simulink model "DeratingControl"  (R2021b)
settings: Solver=VariableStepAuto  StartTime=0.0  StopTime=2  FixedStep=Ts  RelTol=1e-3
model workspace (MAT data in the model file):
  df = Simulink.Parameter
  df.Value = 0.9
  df.DataType = 'auto'
  df.Complexity = 'real'
  df.Dimensions = [1 1]
undefined symbols (not defined in the file or in its folder): const_facInvTempDera, const_facMotTempDera, const_facPwrDera, const_SCD_tqDeraGenOvrd_C, const_stDera, const_tiTaskFast, const_tqBattDeraGenLim, const_tqBattDeraMotLim, const_tqDeraGen, const_tqDeraMot, const_tqDeraMotOvrd_C, const_tqEmMaxNp1, const_tqInvTempDeraMax, const_tqInvTempDeraMin, const_tqMotTempDeraMax, const_tqMotTempDeraMin, const_tqSpLim, const_tqSpLimMax, const_tqSpLimMin, const_tqTqReq
libraries: hdlsllib x10, simulink x4, mcbcontrolslib x1
settings Model: PacingRate=0.350000  Creator=win  LastModifiedBy=win

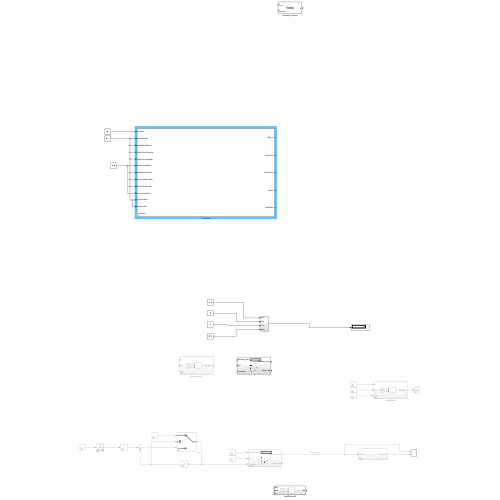
[thumbnail: Simulink's stored preview of the top-level diagram]
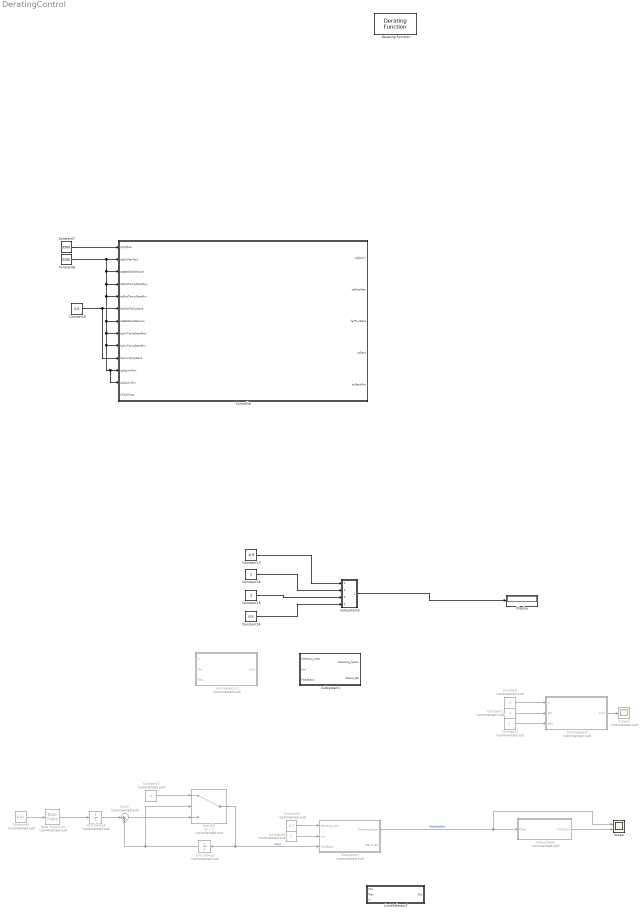
== system DeratingControl ==
  Constant : Constant  Commented=on  Value=-2
  Constant1 : Constant  Commented=on  Value=-1
  Constant13 : Constant  Value=-0.9
  Constant14 : Constant  Value=0.9
  Constant15 : Constant  Value=3
  Constant16 : Constant
  Constant2 : Constant  Commented=on
  Constant3 : Constant  Commented=on  Value=-2
  Constant4 : Constant  Commented=on
  Constant5 : Constant  Commented=on  Value=0.7
  Constant6 : Constant  Commented=on  Value=0.01
  Constant7 : Constant  Value=3500  OutDataTypeStr=int32
  Constant8 : Constant  Value=3200  OutDataTypeStr=int32
  Constant9 : Constant  Value=0.5  OutDataTypeStr=int32
  Controller : Subsystem  Description=Torque setpoint limit maximum value  mask{facGrdLimrUlim_C=50000, facGrdLimrLlim_C=-50000, bDeraMotOvrdActv_C=off, tqDeraMotOvrd_C=0, bDeraGenOvrdActv_C=off, SCD_tqDeraGenOvrd_C=0}
      mask prompts: facGrdLimrUlim_C "Gradient limiter upper factor"; facGrdLimrLlim_C "Gradient limiter lower factor"; bDeraMotOvrdActv_C "Motor mode derating override active"; tqDeraMotOvrd_C "Motor mode derating override torque"; bDeraGenOvrdActv_C "Generator mode derating override active"; SCD_tqDeraGenOvrd_C "Generator mode derating override torque"
  Derating Function : mcbcontrolslib/Derating Function  x=0.9
      settings: SourceProductBaseCode=MT
  Display : Display
  LimitSelector : Subsystem  Commented=on
  LimitSelector1 : Subsystem  Commented=on
  LimitSelector2 : Subsystem
  Rate Transition : RateTransition  Commented=on  OutPortSampleTime=1/36000000
  Scope : Scope  NumInputPorts=2
  Scope1 : Scope  Commented=on
  Subsystem : Subsystem  Commented=on
  Subsystem1 : Subsystem
  Subsystem2 : Subsystem  Commented=on
  Subsystem3 : Subsystem
  Sum1 : Sum  Commented=on  Inputs=|++
  Switch2 : Switch  Commented=on  Criteria=u2 > Threshold  Threshold=2
  Unit Delay2 : UnitDelay  Commented=on  SampleTime=-1  HasFrameUpgradeWarning=on
  Unit Delay3 : UnitDelay  Commented=on  SampleTime=-1  HasFrameUpgradeWarning=on
  wires:
  Unit Delay2/1 -> Switch2/2, Sum1/2
  Constant3/1 -> Switch2/1
  Sum1/1 -> Switch2/3
  Unit Delay3/1 -> Sum1/1
  Switch2/1 -> Subsystem/3(Feedback), Unit Delay2/1  "input"
  Constant4/1 -> Subsystem/2(Lim)
  Constant5/1 -> Subsystem/1(Derating_ratio)
  Subsystem/1(Derating_factor) -> Scope/1, Subsystem2/1(Ratio)  "DeratingOut"
  Subsystem2/1(PWM_Out) -> Scope/2
  Constant6/1 -> Rate Transition/1
  Rate Transition/1 -> Unit Delay3/1
  Constant/1 -> LimitSelector/1(In)
  Constant1/1 -> LimitSelector/2(Min)
  Constant2/1 -> LimitSelector/3(Max)
  LimitSelector/1(Limit) -> Scope1/1
  Constant8/1 -> Controller/3(tqBattDeraMotLim), Controller/4("tqMotTempDeraMax "), Controller/5("tqMotTempDeraMin "), Controller/7(tqBattDeraGenLim), Controller/8(tqInvTempDeraMax), Controller/9(tqInvTempDeraMin), Controller/11("tqSpLimMax "), Controller/12("tqSpLimMin "), Controller/2("tqEmMaxNp1 ")
  Constant7/1 -> Controller/1("tqTqReq ")
  Constant14/1 -> Subsystem3/4(Max)
  Constant13/1 -> Subsystem3/1(Min)
  Constant16/1 -> Subsystem3/2(Sat)
  Constant15/1 -> Subsystem3/3(Live)
  Subsystem3/1(Out1) -> Display/1
  Constant9/1 -> Controller/10("facInvTempDera "), Controller/6("facMotTempDera ")

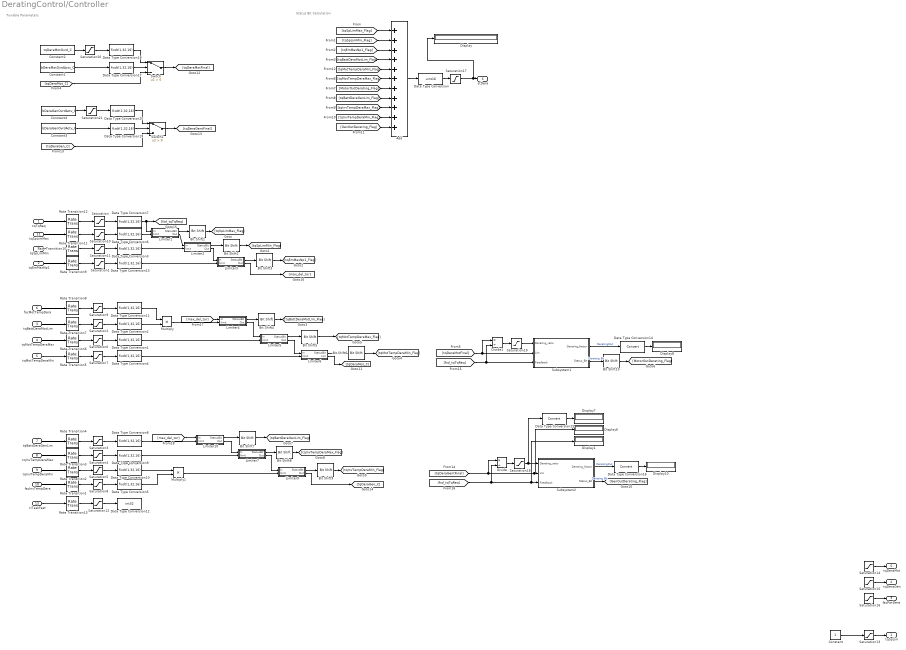
== system DeratingControl/Controller ==
  note: Tunable Parameters
  note: Status Bit Calculation
  "tqTqReq " : Inport  Description=Torque request  OutMin=const_tqTqReq(1)  OutMax=const_tqTqReq(2)  OutDataTypeStr=int32
  "tqEmMaxNp1 " : Inport  Description=EM Maximum torque N+1 step  Port=2  OutMin=const_tqEmMaxNp1(1)  OutMax=const_tqEmMaxNp1(2)  OutDataTypeStr=int32
  tqBattDeraMotLim : Inport  Description=Derated motor mode torque output according to battery limits  Port=3  OutMin=const_tqBattDeraMotLim(1)  OutMax=const_tqBattDeraMotLim(2)  OutDataTypeStr=int32
  "tqMotTempDeraMax " : Inport  Description=Derated torque maximum value according to motor temperature  Port=4  OutMin=const_tqMotTempDeraMax(1)  OutMax=const_tqMotTempDeraMax(2)  OutDataTypeStr=int32
  "tqMotTempDeraMin " : Inport  Description=Derated torque minimum value according to motor temperature  Port=5  OutMin=const_tqMotTempDeraMin(1)  OutMax=const_tqMotTempDeraMin(2)  OutDataTypeStr=int32
  "facMotTempDera " : Inport  Description=Torque derating factor according to motor temperature  Port=6  OutMin=const_facMotTempDera(1)  OutMax=const_facMotTempDera(2)  OutDataTypeStr=int32
  tqBattDeraGenLim : Inport  Description=Derated generator mode torque output according to battery limits  Port=7  OutMin=const_tqBattDeraGenLim(1)  OutMax=const_tqBattDeraGenLim(2)  OutDataTypeStr=int32
  tqInvTempDeraMax : Inport  Description=Derated torque maximum value according to inverter temperature  Port=8  OutMin=const_tqInvTempDeraMax(1)  OutMax=const_tqInvTempDeraMax(2)  OutDataTypeStr=int32
  tqInvTempDeraMin : Inport  Description=Derated torque minimum value according to inverter temperature  Port=9  OutMin=const_tqInvTempDeraMin(1)  OutMax=const_tqInvTempDeraMin(2)  OutDataTypeStr=int32
  "facInvTempDera " : Inport  Description=Torque derating factor according to inverter temperature  Port=10  OutMin=const_facInvTempDera(1)  OutMax=const_facInvTempDera(2)  OutDataTypeStr=int32
  "tqSpLimMax " : Inport  Description=Torque setpoint limit maximum value  Port=11  OutMin=const_tqSpLimMax(1)  OutMax=const_tqSpLimMax(2)  OutDataTypeStr=int32
  "tqSpLimMin " : Inport  Description=Torque setpoint limit minimum value  Port=12  OutMin=const_tqSpLimMin(1)  OutMax=const_tqSpLimMin(2)  OutDataTypeStr=int32
  "tiTaskFast " : Inport  Description=Time for the fast task (PWM task)  Port=13  OutMin=const_tiTaskFast(1)  OutMax=const_tiTaskFast(2)  OutDataTypeStr=int32
  Add : Sum  Inputs=+++++++++++
  Bit Shift1 : hdlsllib/Logic and Bit Operations/Bit Shift  mode=Shift Left Logical  N=0
  Bit Shift10 : hdlsllib/Logic and Bit Operations/Bit Shift  mode=Shift Left Logical  N=6
  Bit Shift2 : hdlsllib/Logic and Bit Operations/Bit Shift  mode=Shift Left Logical  N=1
  Bit Shift3 : hdlsllib/Logic and Bit Operations/Bit Shift  mode=Shift Left Logical  N=2
  Bit Shift4 : hdlsllib/Logic and Bit Operations/Bit Shift  mode=Shift Left Logical  N=3
  Bit Shift5 : hdlsllib/Logic and Bit Operations/Bit Shift  mode=Shift Left Logical  N=4
  Bit Shift6 : hdlsllib/Logic and Bit Operations/Bit Shift  mode=Shift Left Logical  N=5
  Bit Shift7 : hdlsllib/Logic and Bit Operations/Bit Shift  mode=Shift Left Logical  N=7
  Bit Shift8 : hdlsllib/Logic and Bit Operations/Bit Shift  mode=Shift Left Logical  N=8
  Bit Shift9 : hdlsllib/Logic and Bit Operations/Bit Shift  mode=Shift Left Logical  N=9
  Constant : Constant
  Constant1 : Constant  Value=bDeraMotOvrdActv_C
  Constant2 : Constant  Value=tqDeraMotOvrd_C
  Constant3 : Constant  Value=bDeraGenOvrdActv_C
  Constant4 : Constant  Value=bDeraGenOvrdActv_C
  Data Type Conversion : DataTypeConversion  OutDataTypeStr=uint16
  Data Type Conversion{1..11,13,17..20} (16 alike) : DataTypeConversion  OutDataTypeStr=fixdt(1,32,16)
  Data Type Conversion12 : DataTypeConversion  OutDataTypeStr=int32
  Data Type Conversion14 : DataTypeConversion
  Data Type Conversion15 : DataTypeConversion
  Data Type Conversion16 : DataTypeConversion
  Display{,1,6..8,10} (6 alike) : Display
      Display settings: Format=binary (Stored Integer)
  Divide : Product  Inputs=*/  OutDataTypeStr=fixdt(1,32,16)
  Divide1 : Product  Inputs=*/  OutDataTypeStr=fixdt(1,32,16)
  Limiter1 : Subsystem
  Limiter10 : Subsystem
  Limiter2 : Subsystem
  Limiter3 : Subsystem
  Limiter4 : Subsystem
  Limiter5 : Subsystem
  Limiter6 : Subsystem
  Limiter7 : Subsystem
  Limiter9 : Subsystem
  Multiply : Product  Inputs=**
  Multiply1 : Product  Inputs=**
  Rate Transition{1..13} (13 alike) : RateTransition  OutPortSampleTime=Ts
  Saturation : Saturate  UpperLimit=const_tqTqReq(2)  LowerLimit=const_tqTqReq(1)
  Saturation1 : Saturate  UpperLimit=const_tqEmMaxNp1(2)  LowerLimit=const_tqEmMaxNp1(1)
  Saturation10 : Saturate  UpperLimit=const_tqSpLimMax(2)  LowerLimit=const_tqSpLimMax(1)  OutDataTypeStr=int32
  Saturation11 : Saturate  UpperLimit=const_tqSpLimMin(2)  LowerLimit=const_tqSpLimMin(1)  OutDataTypeStr=int32
  Saturation12 : Saturate  UpperLimit=const_tiTaskFast(2)  LowerLimit=const_tiTaskFast(1)  OutDataTypeStr=int32
  Saturation13 : Saturate  UpperLimit=const_tqSpLim(2)  LowerLimit=const_tqSpLim(1)  OutDataTypeStr=int32
  Saturation14 : Saturate  UpperLimit=const_tqDeraMot(2)  LowerLimit=const_tqDeraMot(1)
  Saturation15 : Saturate  UpperLimit=const_tqDeraGen(2)  LowerLimit=const_tqDeraGen(1)
  Saturation16 : Saturate  UpperLimit=const_facPwrDera(2)  LowerLimit=const_facPwrDera(1)
  Saturation17 : Saturate  UpperLimit=const_stDera(2)  LowerLimit=const_stDera(1)  OutDataTypeStr=uint16
  Saturation18 : Saturate  UpperLimit=1  LowerLimit=0  OutDataTypeStr=fixdt(1,32,16)
  Saturation19 : Saturate  UpperLimit=1  LowerLimit=0  OutDataTypeStr=fixdt(1,32,16)
  Saturation2 : Saturate  UpperLimit=const_tqBattDeraMotLim(2)  LowerLimit=const_tqBattDeraMotLim(1)
  Saturation20 : Saturate  UpperLimit=const_tqDeraMotOvrd_C(2)  LowerLimit=const_tqDeraMotOvrd_C(1)  OutDataTypeStr=int32
  Saturation21 : Saturate  UpperLimit=const_SCD_tqDeraGenOvrd_C(2)  LowerLimit=const_SCD_tqDeraGenOvrd_C(1)  OutDataTypeStr=int32
  Saturation3 : Saturate  UpperLimit=const_tqBattDeraGenLim(2)  LowerLimit=const_tqBattDeraGenLim(1)
  Saturation4 : Saturate  UpperLimit=const_tqInvTempDeraMax(2)  LowerLimit=const_tqInvTempDeraMax(1)  OutDataTypeStr=int32
  Saturation5 : Saturate  UpperLimit=const_tqInvTempDeraMin(2)  LowerLimit=const_tqInvTempDeraMin(1)  OutDataTypeStr=int32
  Saturation6 : Saturate  UpperLimit=const_tqMotTempDeraMax(2)  LowerLimit=const_tqMotTempDeraMax(1)  OutDataTypeStr=int32
  Saturation7 : Saturate  UpperLimit=const_tqMotTempDeraMin(2)  LowerLimit=const_tqMotTempDeraMin(1)  OutDataTypeStr=int32
  Saturation8 : Saturate  UpperLimit=1  LowerLimit=0  OutDataTypeStr=int32
  Saturation9 : Saturate  UpperLimit=const_facMotTempDera(2)  LowerLimit=const_facMotTempDera(1)  OutDataTypeStr=int32
  Subsystem1 : Subsystem
  Subsystem2 : Subsystem
  Switch : Switch  Criteria=u2 > Threshold  OutDataTypeStr=fixdt(1,32,16)
  Switch1 : Switch  Criteria=u2 > Threshold  OutDataTypeStr=fixdt(1,32,16)
  "tqSpLim " : Outport  Description=Limited torque setpoint  OutMin=const_tqSpLim(1)  OutMax=const_tqSpLim(2)
  "tqDeraGen " : Outport  Description=Derated torque for generator mode  Port=2  OutMin=const_tqDeraGen(1)  OutMax=const_tqDeraGen(2)
  "facPwrDera " : Outport  Description=Power derating factor  Port=3  OutMin=const_facPwrDera(1)  OutMax=const_facPwrDera(2)
  "stDera " : Outport  Description=Derating status  Port=4  OutMin=const_stDera(1)  OutMax=const_stDera(2)  OutDataTypeStr=uint16
  "tqDeraMot " : Outport  Description=Derated torque for motor mode  Port=5  OutMin=const_tqDeraMot(1)  OutMax=const_tqDeraMot(2)
  wires:
  "tqEmMaxNp1 "/1 -> Rate Transition9/1
  tqBattDeraMotLim/1 -> Rate Transition7/1
  tqBattDeraGenLim/1 -> Rate Transition4/1
  tqInvTempDeraMax/1 -> Rate Transition3/1
  tqInvTempDeraMin/1 -> Rate Transition2/1
  "tqMotTempDeraMax "/1 -> Rate Transition6/1
  "tqMotTempDeraMin "/1 -> Rate Transition5/1
  "facInvTempDera "/1 -> Rate Transition1/1
  "tqSpLimMax "/1 -> Rate Transition11/1
  "tqSpLimMin "/1 -> Rate Transition10/1
  Saturation13/1 -> "tqSpLim "/1
  Saturation15/1 -> "tqDeraGen "/1
  Saturation16/1 -> "facPwrDera "/1
  Saturation17/1 -> Display/1, "stDera "/1
  Saturation6/1 -> Data Type Conversion1/1
  Saturation7/1 -> Data Type Conversion4/1
  Saturation1/1 -> Data Type Conversion13/1
  "facMotTempDera "/1 -> Rate Transition8/1
  Saturation14/1 -> "tqDeraMot "/1
  Saturation9/1 -> Data Type Conversion11/1
  Saturation2/1 -> Data Type Conversion2/1
  Saturation/1 -> Data Type Conversion7/1
  "tqTqReq "/1 -> Rate Transition12/1
  Data Type Conversion13/1 -> Limiter3/2(limit)
  Saturation11/1 -> Data Type Conversion3/1
  Saturation10/1 -> Data Type Conversion6/1
  Data Type Conversion1/1 -> Limiter5/2(limit)
  Data Type Conversion4/1 -> Limiter6/2(limit)
  Data Type Conversion6/1 -> Limiter1/2(limit)
  Data Type Conversion3/1 -> Limiter2/2(limit)
  Limiter2/2(Out) -> Limiter3/1(In)
  Saturation3/1 -> Data Type Conversion8/1
  Saturation4/1 -> Data Type Conversion9/1
  Saturation5/1 -> Data Type Conversion10/1
  Data Type Conversion8/1 -> Limiter10/2(limit)
  Data Type Conversion9/1 -> Limiter7/2(limit)
  Limiter7/2(Out) -> Limiter9/1(In)
  Limiter1/2(Out) -> Limiter2/1(In)
  Limiter5/2(Out) -> Limiter6/1(In)
  Limiter4/2(Out) -> Limiter5/1(In)
  Divide/1 -> Saturation18/1
  Saturation18/1 -> Data Type Conversion15/1, Subsystem2/1(Derating_ratio)
  Divide1/1 -> Saturation19/1
  Saturation19/1 -> Subsystem1/1(Derating_ratio)
  Data Type Conversion2/1 -> Multiply/2
  Data Type Conversion11/1 -> Multiply/1
  Multiply/1 -> Limiter4/2(limit)
  Saturation8/1 -> Data Type Conversion5/1
  Data Type Conversion10/1 -> Multiply1/1
  Data Type Conversion5/1 -> Multiply1/2
  Multiply1/1 -> Limiter9/2(limit)
  Rate Transition1/1 -> Saturation8/1
  Rate Transition2/1 -> Saturation5/1
  Rate Transition3/1 -> Saturation4/1
  Rate Transition4/1 -> Saturation3/1
  Rate Transition5/1 -> Saturation7/1
  Rate Transition6/1 -> Saturation6/1
  Rate Transition7/1 -> Saturation2/1
  Rate Transition8/1 -> Saturation9/1
  Rate Transition9/1 -> Saturation1/1
  Rate Transition10/1 -> Saturation11/1
  Rate Transition11/1 -> Saturation10/1
  Rate Transition12/1 -> Saturation/1
  "tiTaskFast "/1 -> Rate Transition13/1
  Saturation12/1 -> Data Type Conversion12/1
  Rate Transition13/1 -> Saturation12/1
  Limiter1/1(StatusBit) -> Bit Shift1/1
  Limiter10/2(Out) -> Limiter7/1(In)
  Limiter2/1(StatusBit) -> Bit Shift2/1
  Limiter3/1(StatusBit) -> Bit Shift3/1
  Limiter4/1(StatusBit) -> Bit Shift4/1
  Limiter5/1(StatusBit) -> Bit Shift5/1
  Limiter6/1(StatusBit) -> Bit Shift6/1
  Limiter10/1(StatusBit) -> Bit Shift7/1
  Limiter7/1(StatusBit) -> Bit Shift8/1
  Limiter9/1(StatusBit) -> Bit Shift9/1
  Subsystem1/2(Status_Bit) -> Bit Shift10/1  "Derating Bit"
  Bit Shift1/1 -> [tqSpLimMax_Flag]
  Bit Shift2/1 -> [tqSpLimMin_Flag]
  Bit Shift3/1 -> [tqEmMaxNp1_Flag]
  Bit Shift4/1 -> [tqBattDeraMotLim_Flag]
  Bit Shift10/1 -> [MotorOutDerating_Flag]
  Bit Shift7/1 -> [tqBattDeraGenLim_Flag]
  Bit Shift8/1 -> [tqInvTempDeraMax_Flag]
  Bit Shift9/1 -> [tqInvTempDeraMin_Flag]
  Subsystem2/2(Status_Bit) -> [GenOutDerating_Flag]  "Derating Bit"
  [tqSpLimMax_Flag] -> Add/1
  [tqSpLimMin_Flag] -> Add/2
  [tqEmMaxNp1_Flag] -> Add/3
  [tqBattDeraMotLim_Flag] -> Add/4
  Add/1 -> Data Type Conversion/1
  Constant/1 -> Saturation13/1
  Data Type Conversion/1 -> Saturation17/1
  Bit Shift5/1 -> [tqMotTempDeraMax_Flag]
  Bit Shift6/1 -> [tqMotTempDeraMin_Flag]
  [tqMotTempDeraMin_Flag] -> Add/5
  [tqMotTempDeraMax_Flag] -> Add/6
  [MotorOutDerating_Flag] -> Add/7
  [tqBattDeraGenLim_Flag] -> Add/8
  [tqInvTempDeraMax_Flag] -> Add/9
  [tqInvTempDeraMin_Flag] -> Add/10
  [GenOutDerating_Flag] -> Add/11
  Data Type Conversion7/1 -> [fxd_tqTqReq], Limiter1/1(In)
  Subsystem1/1(Derating_factor) -> Data Type Conversion14/1  "DeratingOut"
  Data Type Conversion14/1 -> Display8/1
  Data Type Conversion15/1 -> Display7/1
  Data Type Conversion16/1 -> Display10/1
  Subsystem2/1(Derating_factor) -> Data Type Conversion16/1  "DeratingOut"
  Constant1/1 -> Data Type Conversion17/1
  Data Type Conversion17/1 -> Switch/2
  Saturation20/1 -> Data Type Conversion18/1
  Constant2/1 -> Saturation20/1
  Data Type Conversion18/1 -> Switch/1
  Limiter6/2(Lim) -> [tqDeraMot_C]
  [tqDeraMot_C] -> Switch/3
  Switch/1 -> [tqDeraMotFinal]
  [tqDeraMotFinal] -> Divide1/1, Subsystem1/2(Lim)
  [tqDeraGen_C] -> Switch1/3
  Constant3/1 -> Data Type Conversion19/1
  Switch1/1 -> [tqDeraGentFinal]
  Saturation21/1 -> Data Type Conversion20/1
  Data Type Conversion19/1 -> Switch1/2
  Constant4/1 -> Saturation21/1
  Data Type Conversion20/1 -> Switch1/1
  [tqDeraGentFinal] -> Divide/1, Display6/1, Subsystem2/2(Lim)
  Limiter9/2(Out) -> [tqDeraGen_C]
  [fxd_tqTqReq] -> Subsystem1/3(Feedback), Divide1/2
  [fxd_tqTqReq] -> Divide/2, Display1/1, Subsystem2/3(Feedback)
  Limiter3/2(Out) -> [max_del_tor]
  [max_del_tor] -> Limiter4/1(In)
  [max_del_tor] -> Limiter10/1(In)

== system DeratingControl/LimitSelector ==
  In : Inport
  Min : Inport  Port=2
  Max : Inport  Port=3
  Chart : Stateflow chart  TreatAsAtomicUnit=on
  Limit : Outport
  wires:
  In/1 -> Chart/1(In)
  Max/1 -> Chart/2(Max)
  Min/1 -> Chart/3(Min)
  Chart/1(Limit) -> Limit/1

== system DeratingControl/LimitSelector1 ==
  In : Inport
  Min : Inport  Port=2
  Max : Inport  Port=3
  Chart : Stateflow chart  TreatAsAtomicUnit=on
  Limit : Outport
  wires:
  In/1 -> Chart/1(In)
  Max/1 -> Chart/2(Max)
  Min/1 -> Chart/3(Min)
  Chart/1(Limit) -> Limit/1

== system DeratingControl/LimitSelector2 ==
  Min : Inport
  Max : Inport  Port=2
  In : Inport  Port=3
  Chart : Stateflow chart  TreatAsAtomicUnit=on
  Out : Outport
  wires:
  In/1 -> Chart/1(In)
  Max/1 -> Chart/2(Max)
  Min/1 -> Chart/3(Min)
  Chart/1(Limit) -> Out/1

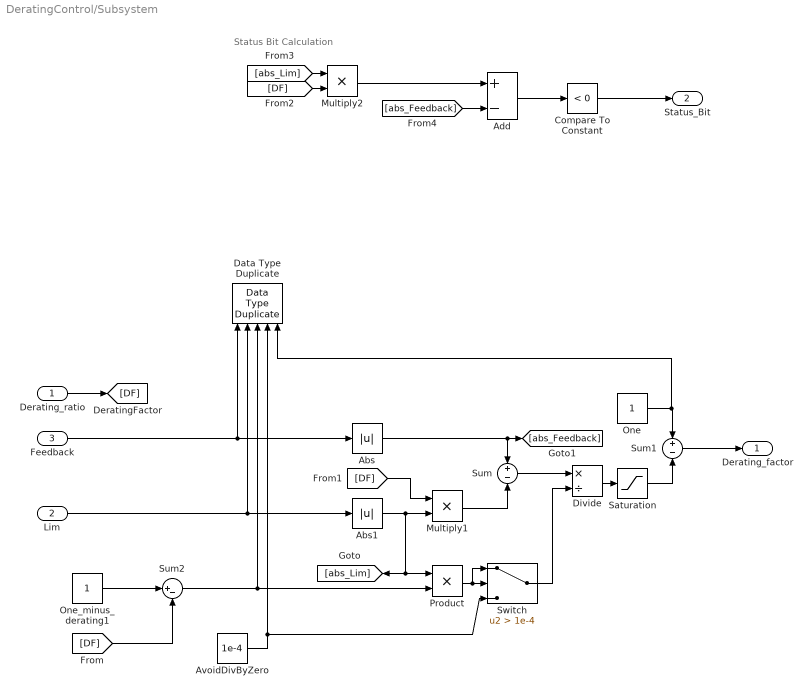
== system DeratingControl/Subsystem ==
  note: Status Bit Calculation
  Derating_ratio : Inport
  Lim : Inport  Port=2
  Feedback : Inport  Port=3
  Abs : Abs  RndMeth=Simplest
  Abs1 : Abs  RndMeth=Simplest
  Add : Sum  Inputs=+-
  AvoidDivByZero : Constant  Value=1e-4  OutDataTypeStr=Inherit: Inherit via back propagation
  Compare To Constant : simulink/Logic and Bit Operations/Compare To Constant  relop=<  const=0  OutDataTypeStr=boolean
  Data Type Duplicate : DataTypeDuplicate  NumInputPorts=5
  Divide : Product  Inputs=*/  RndMeth=Simplest  OutDataTypeStr=Inherit: Same as first input
  Multiply1 : Product  Inputs=**  RndMeth=Simplest  OutDataTypeStr=Inherit: Same as first input
  Multiply2 : Product  Inputs=**  RndMeth=Simplest  OutDataTypeStr=Inherit: Same as first input
  One : Constant  OutDataTypeStr=Inherit: Inherit via back propagation
  One_minus_derating1 : Constant  OutDataTypeStr=Inherit: Inherit via back propagation
  Product : Product  RndMeth=Simplest  OutDataTypeStr=Inherit: Same as first input
  Saturation : Saturate  UpperLimit=1  LowerLimit=0  RndMeth=Simplest
  Sum : Sum  Inputs=+-  RndMeth=Simplest  OutDataTypeStr=Inherit: Same as first input
  Sum1 : Sum  Inputs=+-  RndMeth=Simplest  OutDataTypeStr=Inherit: Same as first input
  Sum2 : Sum  Inputs=|+-
  Switch : Switch  Criteria=u2 > Threshold  Threshold=1e-4
  Derating_factor : Outport  VectorParamsAs1DForOutWhenUnconnected=off
  Status_Bit : Outport  Port=2  OutMin=0  OutMax=1  OutDataTypeStr=boolean  VectorParamsAs1DForOutWhenUnconnected=off
  wires:
  Derating_ratio/1 -> [DF]
  Sum1/1 -> Derating_factor/1
  One/1 -> Sum1/1, Data Type Duplicate/5
  Abs1/1 -> Multiply1/2, Product/1, [abs_Lim]
  Abs/1 -> [abs_Feedback], Sum/1
  Feedback/1 -> Data Type Duplicate/1, Abs/1
  Sum/1 -> Divide/1
  Saturation/1 -> Sum1/2
  Divide/1 -> Saturation/1
  Sum2/1 -> Product/2, Data Type Duplicate/3
  Multiply1/1 -> Sum/2
  Lim/1 -> Abs1/1, Data Type Duplicate/2
  Switch/1 -> Divide/2
  Product/1 -> Switch/1, Switch/2
  AvoidDivByZero/1 -> Data Type Duplicate/4, Switch/3
  [DF] -> Sum2/2
  One_minus_derating1/1 -> Sum2/1
  Add/1 -> Compare To Constant/1
  Compare To Constant/1 -> Status_Bit/1
  [DF] -> Multiply2/2
  Multiply2/1 -> Add/1
  [abs_Lim] -> Multiply2/1
  [abs_Feedback] -> Add/2
  [DF] -> Multiply1/1

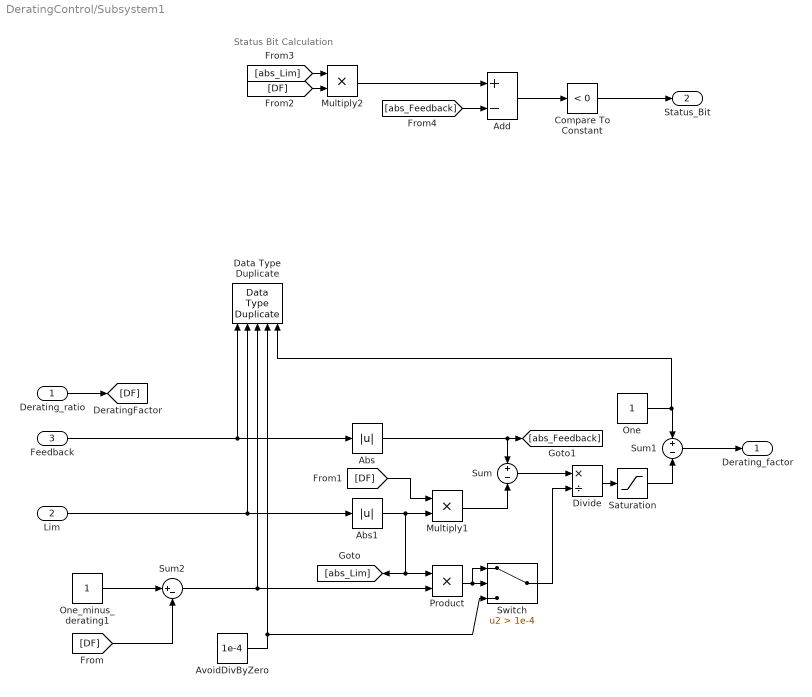
== system DeratingControl/Subsystem1 ==
  note: Status Bit Calculation
  Derating_ratio : Inport
  Lim : Inport  Port=2
  Feedback : Inport  Port=3
  Abs : Abs  RndMeth=Simplest
  Abs1 : Abs  RndMeth=Simplest
  Add : Sum  Inputs=+-
  AvoidDivByZero : Constant  Value=1e-4  OutDataTypeStr=Inherit: Inherit via back propagation
  Compare To Constant : simulink/Logic and Bit Operations/Compare To Constant  relop=<  const=0  OutDataTypeStr=boolean
  Data Type Duplicate : DataTypeDuplicate  NumInputPorts=5
  Divide : Product  Inputs=*/  RndMeth=Simplest  OutDataTypeStr=Inherit: Same as first input
  Multiply1 : Product  Inputs=**  RndMeth=Simplest  OutDataTypeStr=Inherit: Same as first input
  Multiply2 : Product  Inputs=**  RndMeth=Simplest  OutDataTypeStr=Inherit: Same as first input
  One : Constant  OutDataTypeStr=Inherit: Inherit via back propagation
  One_minus_derating1 : Constant  OutDataTypeStr=Inherit: Inherit via back propagation
  Product : Product  RndMeth=Simplest  OutDataTypeStr=Inherit: Same as first input
  Saturation : Saturate  UpperLimit=1  LowerLimit=0  RndMeth=Simplest
  Sum : Sum  Inputs=+-  RndMeth=Simplest  OutDataTypeStr=Inherit: Same as first input
  Sum1 : Sum  Inputs=+-  RndMeth=Simplest  OutDataTypeStr=Inherit: Same as first input
  Sum2 : Sum  Inputs=|+-
  Switch : Switch  Criteria=u2 > Threshold  Threshold=1e-4
  Derating_factor : Outport  VectorParamsAs1DForOutWhenUnconnected=off
  Status_Bit : Outport  Port=2  OutMin=0  OutMax=1  OutDataTypeStr=boolean  VectorParamsAs1DForOutWhenUnconnected=off
  wires:
  [DF] -> Multiply1/1
  [abs_Feedback] -> Add/2
  [abs_Lim] -> Multiply2/1
  Multiply2/1 -> Add/1
  [DF] -> Multiply2/2
  Compare To Constant/1 -> Status_Bit/1
  Add/1 -> Compare To Constant/1
  One_minus_derating1/1 -> Sum2/1
  [DF] -> Sum2/2
  AvoidDivByZero/1 -> Switch/3, Data Type Duplicate/4
  Product/1 -> Switch/2, Switch/1
  Switch/1 -> Divide/2
  Lim/1 -> Data Type Duplicate/2, Abs1/1
  Multiply1/1 -> Sum/2
  Sum2/1 -> Data Type Duplicate/3, Product/2
  Divide/1 -> Saturation/1
  Saturation/1 -> Sum1/2
  Sum/1 -> Divide/1
  Feedback/1 -> Abs/1, Data Type Duplicate/1
  Abs/1 -> Sum/1, [abs_Feedback]
  Abs1/1 -> [abs_Lim], Product/1, Multiply1/2
  One/1 -> Data Type Duplicate/5, Sum1/1
  Sum1/1 -> Derating_factor/1
  Derating_ratio/1 -> [DF]

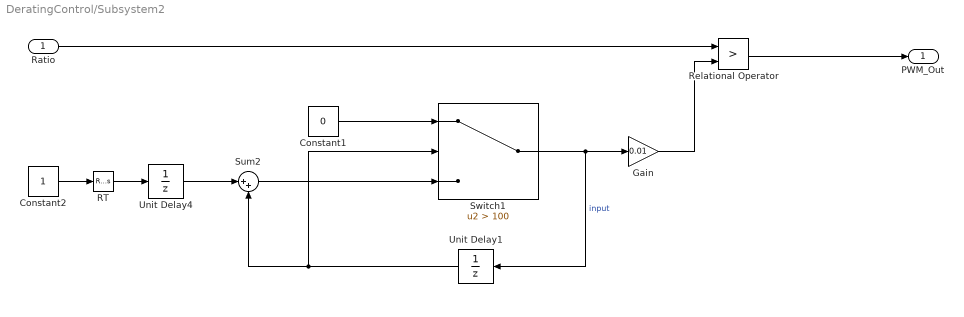
== system DeratingControl/Subsystem2 ==
  Ratio : Inport
  Constant1 : Constant  Value=0
  Constant2 : Constant
  Gain : Gain  Gain=0.01
  RT : RateTransition  Deterministic=off
  Relational Operator : RelationalOperator  Operator=>  OutDataTypeStr=boolean  RndMeth=Simplest
  Sum2 : Sum  Inputs=|++
  Switch1 : Switch  Criteria=u2 > Threshold  Threshold=100
  Unit Delay1 : UnitDelay  SampleTime=-1  HasFrameUpgradeWarning=on
  Unit Delay4 : UnitDelay  SampleTime=-1  HasFrameUpgradeWarning=on
  PWM_Out : Outport
  wires:
  Sum2/1 -> Switch1/3
  Unit Delay1/1 -> Switch1/2, Sum2/2
  Relational Operator/1 -> PWM_Out/1
  Constant2/1 -> RT/1
  Switch1/1 -> Unit Delay1/1, Gain/1  "input"
  Unit Delay4/1 -> Sum2/1
  Ratio/1 -> Relational Operator/1
  RT/1 -> Unit Delay4/1
  Constant1/1 -> Switch1/1
  Gain/1 -> Relational Operator/2

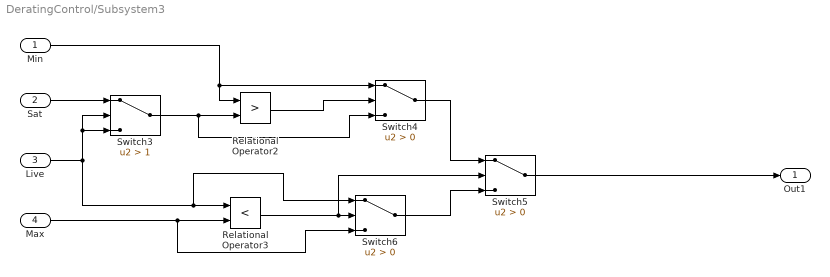
== system DeratingControl/Subsystem3 ==
  Min : Inport
  Sat : Inport  Port=2
  Live : Inport  Port=3
  Max : Inport  Port=4
  Relational Operator2 : RelationalOperator  Operator=>  OutDataTypeStr=boolean  RndMeth=Simplest
  Relational Operator3 : RelationalOperator  Operator=<  OutDataTypeStr=boolean  RndMeth=Simplest
  Switch3 : Switch  Criteria=u2 > Threshold  Threshold=1
  Switch4 : Switch  Criteria=u2 > Threshold
  Switch5 : Switch  Criteria=u2 > Threshold
  Switch6 : Switch  Criteria=u2 > Threshold
  Out1 : Outport
  wires:
  Switch6/1 -> Switch5/3
  Live/1 -> Switch3/3, Switch3/2, Switch6/1, Relational Operator3/1
  Max/1 -> Switch6/3, Relational Operator3/2
  Relational Operator3/1 -> Switch5/2, Switch6/2
  Min/1 -> Relational Operator2/1, Switch4/1
  Switch3/1 -> Switch4/3, Relational Operator2/2
  Relational Operator2/1 -> Switch4/2
  Switch4/1 -> Switch5/1
  Sat/1 -> Switch3/1
  Switch5/1 -> Out1/1

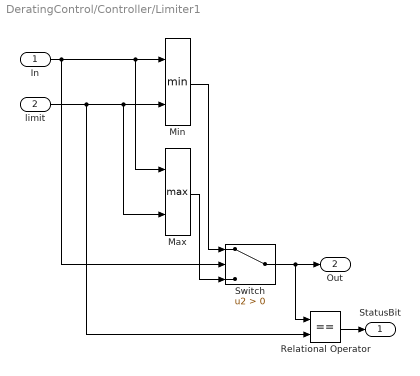
== system DeratingControl/Controller/Limiter1 ==
  In : Inport
  limit : Inport  Port=2
  Max : MinMax  Function=max  Inputs=2
  Min : MinMax  Inputs=2
  Relational Operator : RelationalOperator  Operator===  OutDataTypeStr=fixdt(1,16,0)  RndMeth=Simplest
  Switch : Switch  Criteria=u2 > Threshold
  StatusBit : Outport
  Out : Outport  Port=2
  wires:
  Relational Operator/1 -> StatusBit/1
  Switch/1 -> Out/1, Relational Operator/1
  In/1 -> Switch/2, Max/1, Min/1
  limit/1 -> Max/2, Min/2, Relational Operator/2
  Min/1 -> Switch/1
  Max/1 -> Switch/3

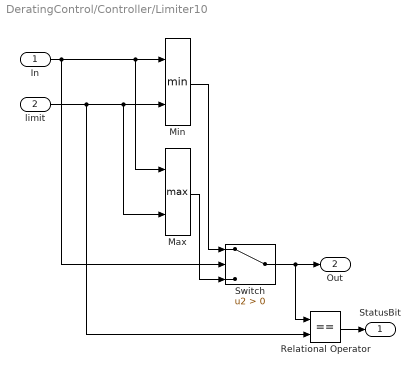
== system DeratingControl/Controller/Limiter10 ==
  In : Inport
  limit : Inport  Port=2
  Max : MinMax  Function=max  Inputs=2
  Min : MinMax  Inputs=2
  Relational Operator : RelationalOperator  Operator===  OutDataTypeStr=fixdt(1,16,0)  RndMeth=Simplest
  Switch : Switch  Criteria=u2 > Threshold
  StatusBit : Outport
  Out : Outport  Port=2
  wires:
  Relational Operator/1 -> StatusBit/1
  Switch/1 -> Out/1, Relational Operator/1
  In/1 -> Switch/2, Max/1, Min/1
  limit/1 -> Max/2, Min/2, Relational Operator/2
  Min/1 -> Switch/1
  Max/1 -> Switch/3

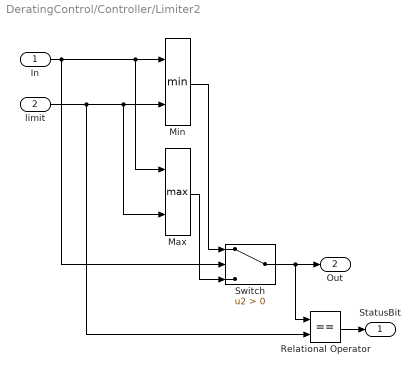
== system DeratingControl/Controller/Limiter2 ==
  In : Inport
  limit : Inport  Port=2
  Max : MinMax  Function=max  Inputs=2
  Min : MinMax  Inputs=2
  Relational Operator : RelationalOperator  Operator===  OutDataTypeStr=fixdt(1,16,0)  RndMeth=Simplest
  Switch : Switch  Criteria=u2 > Threshold
  StatusBit : Outport
  Out : Outport  Port=2
  wires:
  Max/1 -> Switch/3
  Min/1 -> Switch/1
  limit/1 -> Relational Operator/2, Min/2, Max/2
  In/1 -> Min/1, Max/1, Switch/2
  Switch/1 -> Relational Operator/1, Out/1
  Relational Operator/1 -> StatusBit/1

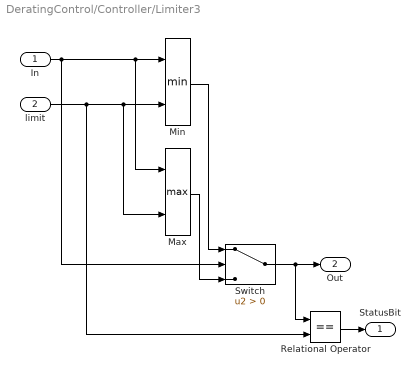
== system DeratingControl/Controller/Limiter3 ==
  In : Inport
  limit : Inport  Port=2
  Max : MinMax  Function=max  Inputs=2
  Min : MinMax  Inputs=2
  Relational Operator : RelationalOperator  Operator===  OutDataTypeStr=fixdt(1,16,0)  RndMeth=Simplest
  Switch : Switch  Criteria=u2 > Threshold
  StatusBit : Outport
  Out : Outport  Port=2
  wires:
  Relational Operator/1 -> StatusBit/1
  Switch/1 -> Out/1, Relational Operator/1
  In/1 -> Switch/2, Max/1, Min/1
  limit/1 -> Max/2, Min/2, Relational Operator/2
  Min/1 -> Switch/1
  Max/1 -> Switch/3

== system DeratingControl/Controller/Limiter4 ==
  In : Inport
  limit : Inport  Port=2
  Max : MinMax  Function=max  Inputs=2
  Min : MinMax  Inputs=2
  Relational Operator : RelationalOperator  Operator===  OutDataTypeStr=fixdt(1,16,0)  RndMeth=Simplest
  Switch : Switch  Criteria=u2 > Threshold
  StatusBit : Outport
  Out : Outport  Port=2
  wires:
  Max/1 -> Switch/3
  Min/1 -> Switch/1
  limit/1 -> Relational Operator/2, Min/2, Max/2
  In/1 -> Min/1, Max/1, Switch/2
  Switch/1 -> Relational Operator/1, Out/1
  Relational Operator/1 -> StatusBit/1

== system DeratingControl/Controller/Limiter5 ==
  In : Inport
  limit : Inport  Port=2
  Max : MinMax  Function=max  Inputs=2
  Min : MinMax  Inputs=2
  Relational Operator : RelationalOperator  Operator===  OutDataTypeStr=fixdt(1,16,0)  RndMeth=Simplest
  Switch : Switch  Criteria=u2 > Threshold
  StatusBit : Outport
  Out : Outport  Port=2
  wires:
  Relational Operator/1 -> StatusBit/1
  Switch/1 -> Out/1, Relational Operator/1
  In/1 -> Switch/2, Max/1, Min/1
  limit/1 -> Max/2, Min/2, Relational Operator/2
  Min/1 -> Switch/1
  Max/1 -> Switch/3

== system DeratingControl/Controller/Limiter6 ==
  In : Inport
  limit : Inport  Port=2
  Max : MinMax  Function=max  Inputs=2
  Min : MinMax  Inputs=2
  Relational Operator : RelationalOperator  Operator===  OutDataTypeStr=fixdt(1,16,0)  RndMeth=Simplest
  Switch : Switch  Criteria=u2 > Threshold
  StatusBit : Outport
  Lim : Outport  Port=2
  wires:
  Max/1 -> Switch/3
  Min/1 -> Switch/1
  limit/1 -> Relational Operator/2, Min/2, Max/2
  In/1 -> Min/1, Max/1, Switch/2
  Switch/1 -> Relational Operator/1, Lim/1
  Relational Operator/1 -> StatusBit/1

== system DeratingControl/Controller/Limiter7 ==
  In : Inport
  limit : Inport  Port=2
  Max : MinMax  Function=max  Inputs=2
  Min : MinMax  Inputs=2
  Relational Operator : RelationalOperator  Operator===  OutDataTypeStr=fixdt(1,16,0)  RndMeth=Simplest
  Switch : Switch  Criteria=u2 > Threshold
  StatusBit : Outport
  Out : Outport  Port=2
  wires:
  Max/1 -> Switch/3
  Min/1 -> Switch/1
  limit/1 -> Relational Operator/2, Min/2, Max/2
  In/1 -> Min/1, Max/1, Switch/2
  Switch/1 -> Relational Operator/1, Out/1
  Relational Operator/1 -> StatusBit/1

== system DeratingControl/Controller/Limiter9 ==
  In : Inport
  limit : Inport  Port=2
  Max : MinMax  Function=max  Inputs=2
  Min : MinMax  Inputs=2
  Relational Operator : RelationalOperator  Operator===  OutDataTypeStr=fixdt(1,16,0)  RndMeth=Simplest
  Switch : Switch  Criteria=u2 > Threshold
  StatusBit : Outport
  Out : Outport  Port=2
  wires:
  Max/1 -> Switch/3
  Min/1 -> Switch/1
  limit/1 -> Relational Operator/2, Min/2, Max/2
  In/1 -> Min/1, Max/1, Switch/2
  Switch/1 -> Relational Operator/1, Out/1
  Relational Operator/1 -> StatusBit/1

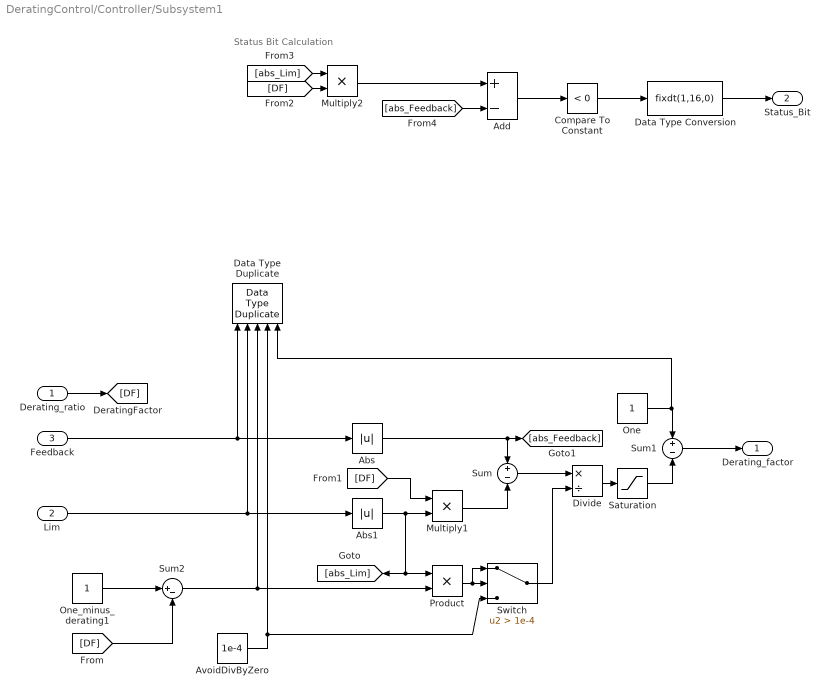
== system DeratingControl/Controller/Subsystem1 ==
  note: Status Bit Calculation
  Derating_ratio : Inport
  Lim : Inport  Port=2
  Feedback : Inport  Port=3
  Abs : Abs  RndMeth=Simplest
  Abs1 : Abs  RndMeth=Simplest
  Add : Sum  Inputs=+-
  AvoidDivByZero : Constant  Value=1e-4  OutDataTypeStr=Inherit: Inherit via back propagation
  Compare To Constant : simulink/Logic and Bit Operations/Compare To Constant  relop=<  const=0  OutDataTypeStr=boolean
  Data Type Duplicate : DataTypeDuplicate  NumInputPorts=5
  Data Type Conversion : DataTypeConversion  OutDataTypeStr=fixdt(1,16,0)
  Divide : Product  Inputs=*/  RndMeth=Simplest  OutDataTypeStr=Inherit: Same as first input
  Multiply1 : Product  Inputs=**  RndMeth=Simplest  OutDataTypeStr=Inherit: Same as first input
  Multiply2 : Product  Inputs=**  RndMeth=Simplest  OutDataTypeStr=Inherit: Same as first input
  One : Constant  OutDataTypeStr=Inherit: Inherit via back propagation
  One_minus_derating1 : Constant  OutDataTypeStr=Inherit: Inherit via back propagation
  Product : Product  RndMeth=Simplest  OutDataTypeStr=Inherit: Same as first input
  Saturation : Saturate  UpperLimit=1  LowerLimit=0  RndMeth=Simplest
  Sum : Sum  Inputs=+-  RndMeth=Simplest  OutDataTypeStr=Inherit: Same as first input
  Sum1 : Sum  Inputs=+-  RndMeth=Simplest  OutDataTypeStr=Inherit: Same as first input
  Sum2 : Sum  Inputs=|+-
  Switch : Switch  Criteria=u2 > Threshold  Threshold=1e-4
  Derating_factor : Outport  VectorParamsAs1DForOutWhenUnconnected=off
  Status_Bit : Outport  Port=2  OutMin=0  OutMax=1  OutDataTypeStr=fixdt(1,16,0)  VectorParamsAs1DForOutWhenUnconnected=off
  wires:
  [DF] -> Multiply1/1
  [abs_Feedback] -> Add/2
  [abs_Lim] -> Multiply2/1
  Multiply2/1 -> Add/1
  [DF] -> Multiply2/2
  Compare To Constant/1 -> Data Type Conversion/1
  Add/1 -> Compare To Constant/1
  One_minus_derating1/1 -> Sum2/1
  [DF] -> Sum2/2
  AvoidDivByZero/1 -> Switch/3, Data Type Duplicate/4
  Product/1 -> Switch/2, Switch/1
  Switch/1 -> Divide/2
  Lim/1 -> Data Type Duplicate/2, Abs1/1
  Multiply1/1 -> Sum/2
  Sum2/1 -> Data Type Duplicate/3, Product/2
  Divide/1 -> Saturation/1
  Saturation/1 -> Sum1/2
  Sum/1 -> Divide/1
  Feedback/1 -> Abs/1, Data Type Duplicate/1
  Abs/1 -> Sum/1, [abs_Feedback]
  Abs1/1 -> [abs_Lim], Product/1, Multiply1/2
  One/1 -> Data Type Duplicate/5, Sum1/1
  Sum1/1 -> Derating_factor/1
  Derating_ratio/1 -> [DF]
  Data Type Conversion/1 -> Status_Bit/1

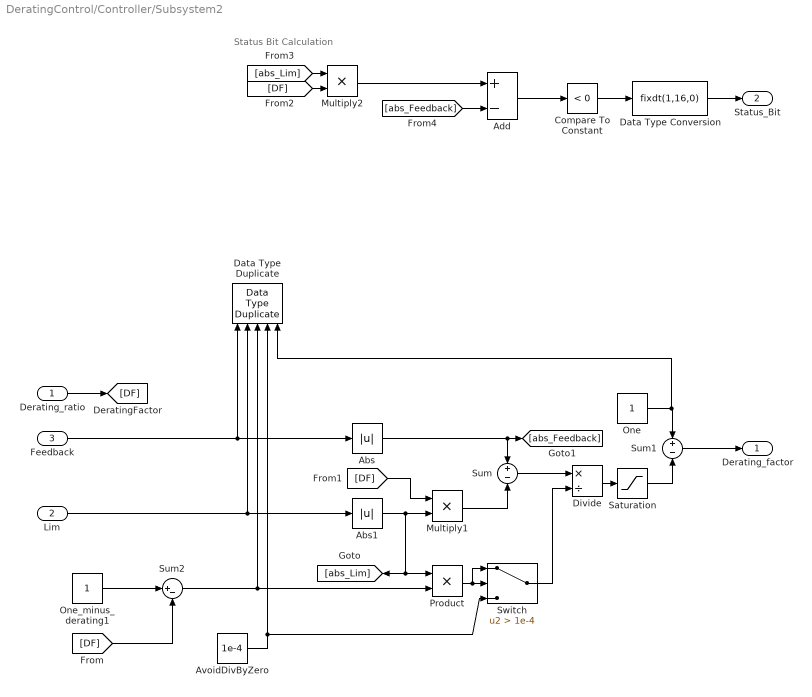
== system DeratingControl/Controller/Subsystem2 ==
  note: Status Bit Calculation
  Derating_ratio : Inport
  Lim : Inport  Port=2
  Feedback : Inport  Port=3
  Abs : Abs  RndMeth=Simplest
  Abs1 : Abs  RndMeth=Simplest
  Add : Sum  Inputs=+-
  AvoidDivByZero : Constant  Value=1e-4  OutDataTypeStr=Inherit: Inherit via back propagation
  Compare To Constant : simulink/Logic and Bit Operations/Compare To Constant  relop=<  const=0  OutDataTypeStr=boolean
  Data Type Duplicate : DataTypeDuplicate  NumInputPorts=5
  Data Type Conversion : DataTypeConversion  OutDataTypeStr=fixdt(1,16,0)
  Divide : Product  Inputs=*/  RndMeth=Simplest  OutDataTypeStr=Inherit: Same as first input
  Multiply1 : Product  Inputs=**  RndMeth=Simplest  OutDataTypeStr=Inherit: Same as first input
  Multiply2 : Product  Inputs=**  RndMeth=Simplest  OutDataTypeStr=Inherit: Same as first input
  One : Constant  OutDataTypeStr=Inherit: Inherit via back propagation
  One_minus_derating1 : Constant  OutDataTypeStr=fixdt(1,32,16)
  Product : Product  RndMeth=Simplest  OutDataTypeStr=Inherit: Same as first input
  Saturation : Saturate  UpperLimit=1  LowerLimit=0  RndMeth=Simplest
  Sum : Sum  Inputs=+-  RndMeth=Simplest  OutDataTypeStr=Inherit: Same as first input
  Sum1 : Sum  Inputs=+-  RndMeth=Simplest  OutDataTypeStr=Inherit: Same as first input
  Sum2 : Sum  Inputs=|+-
  Switch : Switch  Criteria=u2 > Threshold  Threshold=1e-4
  Derating_factor : Outport  VectorParamsAs1DForOutWhenUnconnected=off
  Status_Bit : Outport  Port=2  OutMin=0  OutMax=1  OutDataTypeStr=fixdt(1,16,0)  VectorParamsAs1DForOutWhenUnconnected=off
  wires:
  Derating_ratio/1 -> [DF]
  Sum1/1 -> Derating_factor/1
  One/1 -> Sum1/1, Data Type Duplicate/5
  Abs1/1 -> Multiply1/2, Product/1, [abs_Lim]
  Abs/1 -> [abs_Feedback], Sum/1
  Feedback/1 -> Data Type Duplicate/1, Abs/1
  Sum/1 -> Divide/1
  Saturation/1 -> Sum1/2
  Divide/1 -> Saturation/1
  Sum2/1 -> Product/2, Data Type Duplicate/3
  Multiply1/1 -> Sum/2
  Lim/1 -> Abs1/1, Data Type Duplicate/2
  Switch/1 -> Divide/2
  Product/1 -> Switch/1, Switch/2
  AvoidDivByZero/1 -> Data Type Duplicate/4, Switch/3
  [DF] -> Sum2/2
  One_minus_derating1/1 -> Sum2/1
  Add/1 -> Compare To Constant/1
  Compare To Constant/1 -> Data Type Conversion/1
  [DF] -> Multiply2/2
  Multiply2/1 -> Add/1
  [abs_Lim] -> Multiply2/1
  [abs_Feedback] -> Add/2
  [DF] -> Multiply1/1
  Data Type Conversion/1 -> Status_Bit/1

== stateflow chart DeratingControl/LimitSelector1/Chart ==
  state LimitSelector
    Limit= Max;
  state Min
    Limit=Min;
  (default) -> LimitSelector
  LimitSelector -> Min : [In < Min]
  Min -> LimitSelector : [[In >= Min]]
  data: In input; Max input; Min input; Limit output

== stateflow chart DeratingControl/LimitSelector2/Chart ==
  state LimitSelector
    Limit= Max;
  state Min
    Limit=Min;
  (default) -> LimitSelector
  LimitSelector -> Min : [In < Min]
  Min -> LimitSelector : [[In >= Min]]
  data: In input; Max input; Min input; Limit output

== stateflow chart DeratingControl/LimitSelector/Chart ==
  state LimitSelector
    Limit= Max;
  state Min
    Limit=Min;
  (default) -> LimitSelector
  LimitSelector -> Min : [In < Min]
  Min -> LimitSelector : [[In >= Min]]
  data: In input; Max input; Min input; Limit output
